simulink model "master_arm"  (R2016b)
settings: Solver=ode3  StartTime=0.0  StopTime=inf  RelTol=1e-3  EnableMultiTasking=on
libraries: vexarmcortexlib x3
settings Model: ExtModeTrigDuration=25  Creator=gyanwen  LastModifiedBy=gyanwen
settings DataIOCC: LimitDataPoints=on  SignalLoggingSaveFormat=ModelDataLogs
settings OptimizationCC: ExpressionDepthLimit=2147483647  LifeSpan=Inf  MaxStackSize=64
settings DebuggingCC: UnderspecifiedInitializationDetection=Classic  MergeDetectMultiDrivingBlocksExec=none  InheritedTsInSrcMsg=none  FcnCallInpInsideContextMsg=warning  UnconnectedInputMsg=none  UnconnectedOutputMsg=none  StateNameClashWarn=warning  SFUnexpectedBacktrackingDiag=warning  SFNoUnconditionalDefaultTransitionDiag=warning  SFExecutionAtInitializationDiag=none
settings HardwareCC: ProdBitPerPointer=32  ProdBitPerSizeT=32  ProdBitPerPtrDiffT=32  ProdLargestAtomicInteger=Long  ProdLargestAtomicFloat=Double  ProdIntDivRoundTo=Undefined  ProdWordSize=32  ProdHWDeviceType=ARM Compatible->ARM Cortex
settings ModelReferenceCC: PropagateSignalLabelsOutOfModel=off
settings RTWCC: SystemTargetFile=ert.tlc  HardwareBoard=ARM Cortex-based VEX Microcontroller  TemplateMakefile=ert_default_tmf  Description=Embedded Coder  Toolchain=GNU Tools for VEX ARM Cortex
settings CodeAppCC: IgnoreCustomStorageClasses=off  CustomSymbolStrType=$N$R$M  InternalIdentifier=Classic
settings ERTTargetCC: CodeReplacementLibrary=GCC ARM Cortex-M3  ConvertIfToSwitch=off  SuppressUnreachableDefaultCases=off

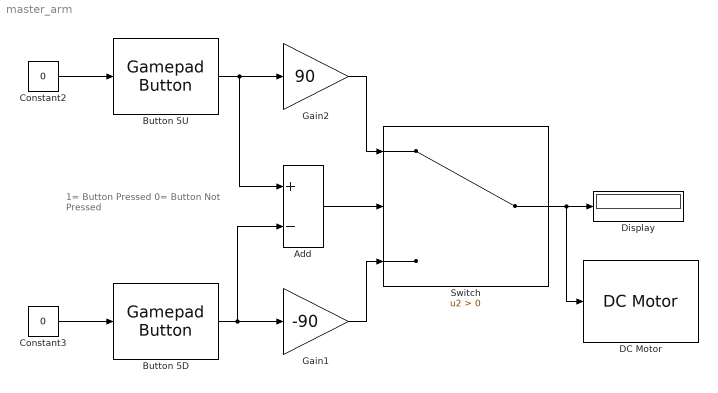
== system master_arm ==
  note: 1= Button Pressed
      | 0= Button Not Pressed
  Add : Sum  Inputs=+-
  Button 5D : vexarmcortexlib/Gamepad Button  joystick=1  chan=5  button56=Down  button78=Right  SimulationIn=on  sample_time=-1
  Button 5U : vexarmcortexlib/Gamepad Button  joystick=1  chan=5  button56=Up  button78=Right  SimulationIn=on  sample_time=-1
  Constant2 : Constant  Value=0
  Constant3 : Constant  Value=0
  DC Motor : vexarmcortexlib/DC Motor  motor=4  scaleFactor=1/13.5  SimulationOut=off
  Display : Display
  Gain1 : Gain  Gain=-90
  Gain2 : Gain  Gain=90
  Switch : Switch  Criteria=u2 > Threshold
  wires:
  Switch/1 -> DC Motor/1, Display/1
  Constant2/1 -> Button 5U/1
  Constant3/1 -> Button 5D/1
  Gain1/1 -> Switch/3
  Gain2/1 -> Switch/1
  Add/1 -> Switch/2
  Button 5U/1 -> Add/1, Gain2/1
  Button 5D/1 -> Add/2, Gain1/1
